simulink model "Pendubot_PFL_LQR"  (R2025b)
settings: Solver=FixedStepAuto  StartTime=0.0  StopTime=Tsim  FixedStep=T  RelTol=1e-3
values from neighbouring files (symbols this model uses):
  K = lqr(A, B, Q, R)    [k_LQR.m]    (also in run_pendubot_simulink.m = k_LQR())
  T = 1e-3    (= 0.001)    [run_pendubot_simulink.m]
  X0 = [-90*pi/180; 0*pi/180; 0; 0]    [run_pendubot_simulink.m]
  xF = [pi/2; 0; 0; 0]    [MAIN.m]    (also in k_LQR.m; run_pendubot_simulink.m)
settings Model: Creator=katiebyl  LastModifiedBy=24573

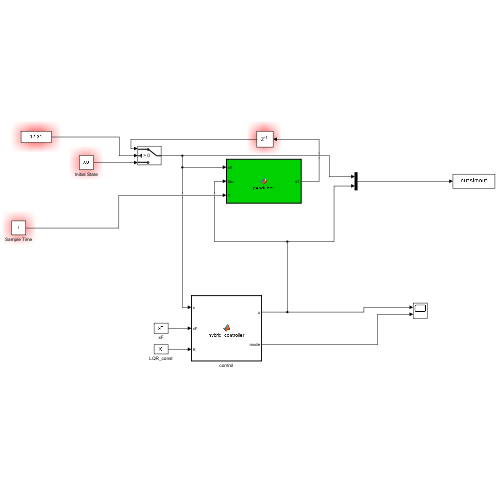
[thumbnail: Simulink's stored preview of the top-level diagram]
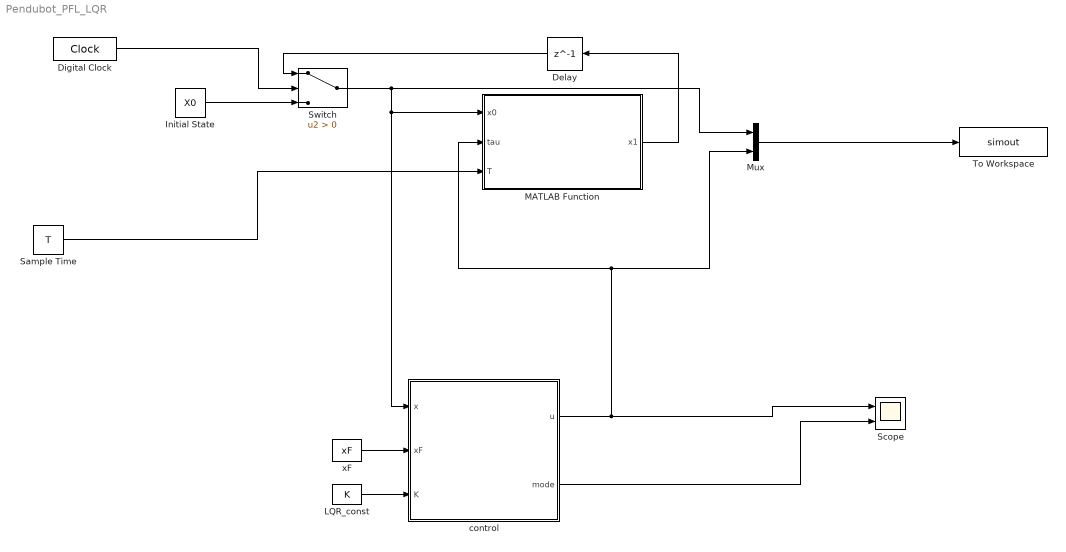
== system Pendubot_PFL_LQR ==
  Delay : Delay  DelayLength=1  InitialCondition=X0
  Digital Clock : DigitalClock  SampleTime=T
  Initial State : Constant  Value=X0
  LQR_const : Constant  Value=K
  MATLAB Function : MATLAB Function  TreatAsAtomicUnit=on
  Mux : Mux  Inputs=2
  Sample Time : Constant  Value=T
  Scope : Scope  NumInputPorts=2
      settings: ActiveDisplayYMinimum=-9.8933  ActiveDisplayYMaximum=9.0082
  Switch : Switch  Criteria=u2 > Threshold  SaturateOnIntegerOverflow=off  InputSameDT=off
  To Workspace : ToWorkspace  VariableName=simout  SaveFormat=Timeseries  SampleTime=-1
  control : MATLAB Function  TreatAsAtomicUnit=on
  xF : Constant  Value=xF
  wires:
  Sample Time/1 -> MATLAB Function/3(T)
  MATLAB Function/1(x1) -> Delay/1
  Initial State/1 -> Switch/3
  Delay/1 -> Switch/1
  Digital Clock/1 -> Switch/2
  Switch/1 -> MATLAB Function/1(x0), control/1(x), Mux/1
  Mux/1 -> To Workspace/1
  LQR_const/1 -> control/3(K)
  control/1(u) -> Scope/1, MATLAB Function/2(tau), Mux/2
  control/2(mode) -> Scope/2
  xF/1 -> control/2(xF)

== matlab function Pendubot_PFL_LQR/control ==
  data: x input; xF input; K input; u output size=1; mode output
function [u, mode] = hybrid_controller(x, xF, K)
    u_max = 12;
    uF=0; kp = 4250;kd = 180;
    persistent lqr_engaged;
    if isempty(lqr_engaged)
        lqr_engaged = false;
    end
    % 1. Calculate Error
    error = x(1:4) - xF(1:4);
    
    % 2. Define Switching Condition
    e_pos = atan2(sin(error(1:2)), cos(error(1:2)));
    pos_err = norm(e_pos);
    e_vel = error(3:4);
    vel_err = norm(e_vel);

    %disp(error)
    if ((pos_err >= 0.8) || (vel_err >= 20.0)) && (lqr_engaged == false)
        % --- SWING UP MODE (Trajectory Playback) ---
        mode = 0;
        u = pendubot_pfl_controller(x(1:4), xF(1), xF(3), uF, kp, kd);
        %disp('PFL Activated');
        % disp(mode);
    else
        lqr_engaged = true;
        % --- LQR MODE ---
        mode = 1;
        x_error = [e_pos; e_vel];
        x_error = x_error(1:4, 1);
        K= K';
        v = -K(1,1:4)*x_error;
        u = inverse_dynamics_pfl(x,v);
        u = u(1);
        % disp('LQR Activated');
    end
    
    % 3. Saturation (Physical Limits)
    u = max(min(u, u_max), -u_max);
    % disp(mode);
end

% --- PFL Helper: Calculates dynamics assuming q1_ddot = v ---
function dx = pfl_virtual_dynamics(x, v)
    % Unpack
    q1 = x(1); q2 = x(2); dq1 = x(3); dq2 = x(4);
    
    % Get Matrices
    [D, H, Phi] = get_matrices(x);
    d21 = D(2,1); d22 = D(2,2);
    h2 = H(2); phi2 = Phi(2);
    
    % If we force ddq1 = v, what happens to ddq2?
    % Equation 2: d21*v + d22*ddq2 + h2 + phi2 = 0
    % ddq2 = -inv(d22) * (d21*v + h2 + phi2)
    
    ddq2 = -(d21*v + h2 + phi2) / d22;
    
    dx = [dq1; dq2; v; ddq2];
end

% --- PFL Helper: Calculates Torque to achieve q1_ddot = v ---
function tau = inverse_dynamics_pfl(x, v)
    % Unpack
    % q1 = x(1); q2 = x(2); dq1 = x(3); dq2 = x(4);
    
    [D, H, Phi] = get_matrices(x);
    d11 = D(1,1); d12 = D(1,2);
    d21 = D(2,1); d22 = D(2,2);
    h1 = H(1); h2 = H(2);
    phi1 = Phi(1); phi2 = Phi(2);
    
    % From PFL derivation (Collocated Linearization):
    % tau = M_bar * v + N_bar
    
    % M_bar = d11 - d12*inv(d22)*d21
    m_bar = d11 - (d12 * d21 / d22);
    
    % N_bar = (h1 + phi1) - d12*inv(d22)*(h2 + phi2)
    n_bar = (h1 + phi1) - (d12 / d22) * (h2 + phi2);
    
    tau = m_bar * v + n_bar;
end

% --- Standard Matrices Helper ---
function [D, H, Phi] = get_matrices(x)
    q1 = x(1); q2 = x(2); dq1 = x(3); dq2 = x(4);
    
    g   = 9.81;
    Th1 = 3.08e-2; Th2 = 1.06e-2; Th3 = 9.5e-3;
    Th4 = 2.087e-1; Th5 = 6.3e-2;
    
    c2 = cos(q2); s2 = sin(q2);
    c1 = cos(q1); c12 = cos(q1+q2);

    D = [Th1 + Th2 + 2*Th3*c2,  Th2 + Th3*c2;
         Th2 + Th3*c2,          Th2];
     
    h_term = Th3 * s2;
    H = [-h_term * dq2 * (2*dq1 + dq2);
          h_term * dq1^2];
      
    Phi = [Th4*g*c1 + Th5*g*c12;
           Th5*g*c12];
end

%%pfl

function tau = pendubot_pfl_controller(x, q1d, dq1d, ddq1d, kp, kd)

% x = [q1;q2;dq1;dq2]
q1  = x(1);  q2  = x(2);
dq1 = x(3);  dq2 = x(4);

% Parameters (must match pendubot_dynamics.m)
g  = 9.8;
Th1 = 3.08e-2;
Th2 = 1.06e-2;
Th3 = 9.5e-3;
Th4 = 2.087e-1;
Th5 = 6.3e-2;

cosq1 = cos(q1);
cosq2 = cos(q2);
sinq2 = sin(q2);
cosq1q2 = cos(q1+q2);

% Inertia terms (same as dynamics file)
d11 = Th1 + Th2 + 2*Th3*cosq2;
d12 = Th2 + Th3*cosq2;
d22 = Th2;

% Coriolis/centrifugal terms
h1 = -Th3*sinq2*dq2*(dq1+dq2);
h2 =  Th3*sinq2*dq1^2;

% Gravity terms
phi1 = Th4*g*cosq1 + Th5*g*cosq1q2;
phi2 = Th5*g*cosq1q2;

% PFL scalars
Delta = d11 - (d12^2)/d22;
beta  = (h1 + phi1) - (d12/d22)*(h2 + phi2);

% Virtual input v to impose ddq1 = v
v = ddq1d - kd*(dq1 - dq1d) - kp*(q1 - q1d);

% Shoulder torque
tau = Delta*v + beta;

end

== matlab function Pendubot_PFL_LQR/MATLAB Function ==
  data: x0 input; x1 output; tau input; T input
function x1 = pendubot(x0, tau, T)

% function x1 = pendubot(x0)
%
% This function simulates the nonlinear dynamics of the
% pendubot on a discrete-time basis. 
%   input:  x0 is x(k)
%   output: x1 is x(k+1)
%
% The parameters are from the Pendubot manual, on the
% canvas page for "Final Project / Pendubot".
%
% Katie Byl, UCSB, ECE 238

% T = 1e-3; % Sample Time (s) - needs to match rest of model
g = 9.81; % gravity (m/(s^2))

Th1 = 3.08e-2;
Th2 = 1.06e-2;
Th3 = 9.5e-3;
Th4 = 2.087e-1;
Th5 = 6.3e-2;

q1 = x0(1); q2 = x0(2); % encoder angles, in radians
dq1 = x0(3); dq2 = x0(4); % angular velocities (rad/s)

cosq1 = cos(q1);
cosq2 = cos(q2); 
sinq2 = sin(q2);
cosq1q2 = cos(q1+q2);

d11 = Th1 + Th2 + 2 * Th3 * cosq2;
d12 = Th2 + Th3 * cosq2;
d22 = Th2;
D = [d11 d12; d12 d22];

h1 = -Th3 * sinq2 * dq2 * (dq1+dq2);
h2 = Th3 * sinq2 * dq1^2;
H = [h1; h2];

phi1 = Th4 * g * cosq1 + Th5 * g * cosq1q2;
phi2 = Th5 * g * cosq1q2;
Phi = [phi1; phi2];

Tau = [tau; 0]; % torque (N*m) applied to first link

%% Equation on motion, in matrix form, is:
%     D*d2q + H + Phi = [tau; 0] = Tau
%  (i.e., tau is applied at the FIRST link, for the pendubot)
%
%  Rearranging, we get:
%     D*d2q = Tau - H - Phi
%  which can be solved via the backslash:
%       d2q = D \ (Tau - H - Phi)

d2q = D \ (Tau - H - Phi);
dX = [x0(3:4); d2q]; % velocities and accelerations

% For "small T", we can use forward Euler to approximate
% the dynamics:

x1 = x0 + T*dX;  % forward Euler integration

%% End of function
